simulink model "Voltage_PI"  (R2020a)
settings: Solver=VariableStepAuto  StartTime=0.0  StopTime=0.2  RelTol=1e-3
values from neighbouring files (symbols this model uses):
  Ki_v = Kp_v * wc_v    (= 1666.66666667)    [parameter.m]
  Kp_v = Gain_v * 5    (= 5)    [parameter.m]
settings Model: Creator=ykamatan  LastModifiedBy=ykamatan
settings SolverCC: ZeroCrossAlgorithm=Adaptive
settings DataIOCC: SaveOutput=off  SaveTime=off
settings DebuggingCC: IgnoredZcDiagnostic=none

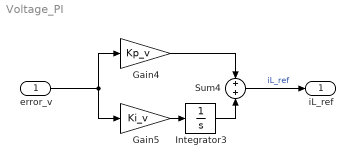
== system Voltage_PI ==
  error_v : Inport  OutDataTypeStr=double  PortDimensions=1  SampleTime=[5.0000000000000004e-06,0]
  Gain4 : Gain  Gain=Kp_v
  Gain5 : Gain  Gain=Ki_v
  Integrator3 : Integrator
  Sum4 : Sum  Inputs=+|+
  iL_ref : Outport  OutDataTypeStr=double  PortDimensions=1  SampleTime=0
  wires:
  error_v/1 -> Gain4/1, Gain5/1
  Gain5/1 -> Integrator3/1
  Gain4/1 -> Sum4/1
  Integrator3/1 -> Sum4/2
  Sum4/1 -> iL_ref/1  "iL_ref"
